simulink model "breath_test"  (R2026a)
settings: Solver=ode23t  StopTime=60*60  MaxStep=0.1  RelTol=1e-4
libraries: fl_lib x3
settings Model: DataDictionary=scubaParams.sldd  Creator=grouleau  LastModifiedBy=grouleau
settings SimscapeCC: SimscapeLogType=none  SimscapeLogOpenViewer=on

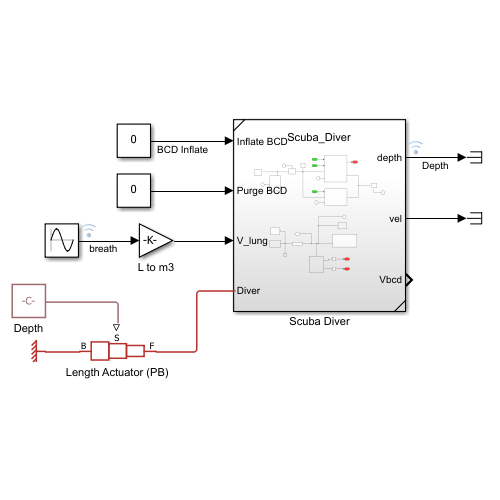
[thumbnail: Simulink's stored preview of the top-level diagram]
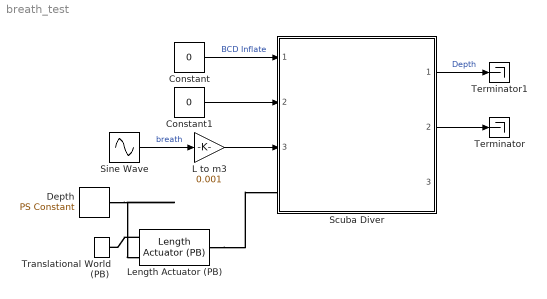
== system breath_test ==
  Constant : Constant  Value=0
  Constant1 : Constant  Value=0
  Depth : fl_lib/Physical Signals/Sources/PS Constant  constant=breathTestDepth m
  L to m3 : Gain  Gain=0.001
  Length Actuator (PB) : fl_lib/Translational/Sources/Length Actuator (PB)  f_specify=off  f_priority=None  f=0 N  f_nominal_specify=off  f_nominal_value=1  f_nominal_unit=N  v_rel_specify=off  v_rel_priority=None  v_rel=0 m/s  v_rel_nominal_specify=off  v_rel_nominal_value=1  v_rel_nominal_unit=m/s  length_specify=off  length_priority=None  length=0 m  length_nominal_specify=off  length_nominal_value=1  length_nominal_unit=m
  Scuba Diver : Subsystem  ReferencedSubsystem=Scuba_Diver
  Sine Wave : Sin  Amplitude=0.5  Bias=2.75  Frequency=0.1*2*pi  SampleTime=0
  Terminator : Terminator
  Terminator1 : Terminator
  Translational World (PB) : fl_lib/Translational/Elements/Translational World (PB)
  wires:
  Scuba Diver/1 -> Terminator1/1  "Depth"
  Constant/1 -> Scuba Diver/1  "BCD Inflate"
  Constant1/1 -> Scuba Diver/2
  Scuba Diver/2 -> Terminator/1
  Sine Wave/1 -> L to m3/1  "breath"
  L to m3/1 -> Scuba Diver/3
  connections:
  Length Actuator (PB)/LConn1 -- Translational World (PB)/RConn1
  Length Actuator (PB)/RConn1 -- Scuba Diver/LConn1
  Depth/RConn1 -- Length Actuator (PB)/LConn2
